simulink model "Tema_bonus_Pisai_Daria_PC1"  (R2024b)
settings: Solver=FixedStepAuto  StartTime=0.0  StopTime=1000  FixedStep=0.01  RelTol=1e-3
settings Model: Creator=dariapisai  LastModifiedBy=dariapisai

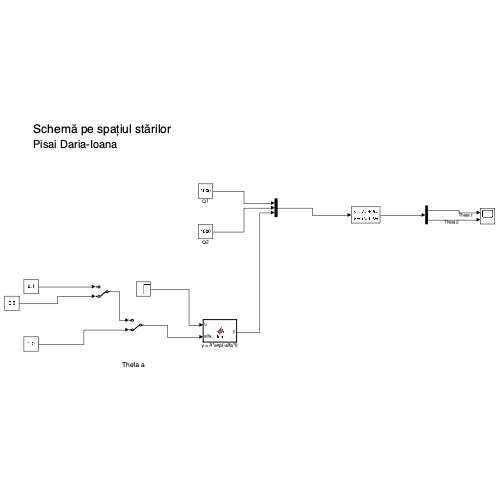
[thumbnail: Simulink's stored preview of the top-level diagram]
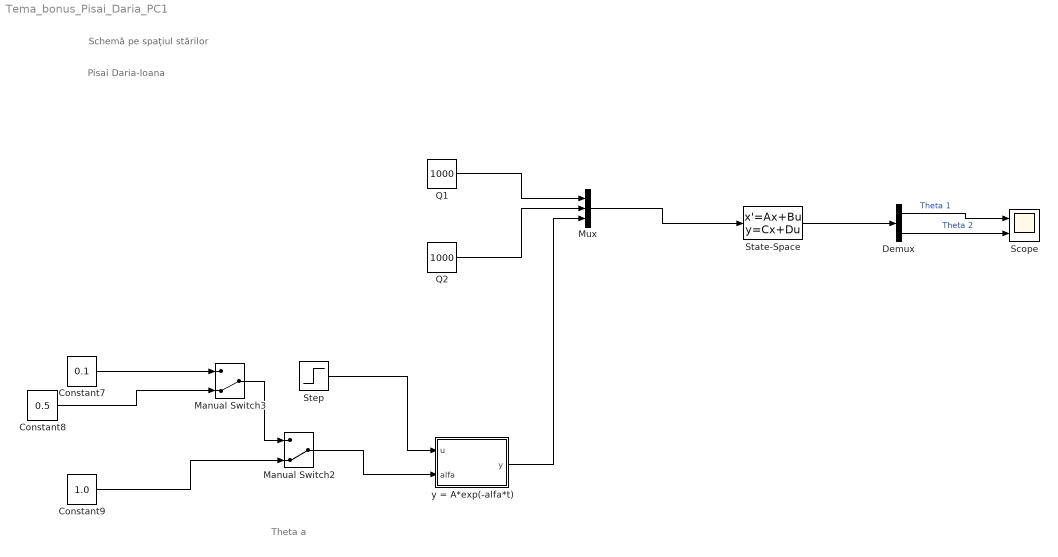
== system Tema_bonus_Pisai_Daria_PC1 ==
  note: Pisai Daria-Ioana
  note: Schemă pe spațiul stărilor
  note: Theta a
  Constant7 : Constant  Value=0.1
  Constant8 : Constant  Value=0.5
  Constant9 : Constant  Value=1.0
  Demux : Demux  Outputs=2
  Manual Switch2 : ManualSwitch  CurrentSetting=0
  Manual Switch3 : ManualSwitch  CurrentSetting=0
  Mux : Mux  Inputs=3
  Q1 : Constant  Value=1000
  Q2 : Constant  Value=1000
  Scope : Scope  NumInputPorts=2
  State-Space : StateSpace  A=[-3/625 1/1250; 1/1500 -1/1000]  B=[1/250 0 1/250; 0 1/300 1/3000]  C=[1 0; 0 1]  D=[0 0 0; 0 0 0]  InitialCondition=0
  Step : Step  Time=5  SampleTime=0
  y = A*exp(-alfa*t) : MATLAB Function  TreatAsAtomicUnit=on
  wires:
  Q1/1 -> Mux/1
  Q2/1 -> Mux/2
  Mux/1 -> State-Space/1
  Constant9/1 -> Manual Switch2/2
  Constant8/1 -> Manual Switch3/2
  Manual Switch3/1 -> Manual Switch2/1
  y = A*exp(-alfa*t)/1(y) -> Mux/3
  Manual Switch2/1 -> y = A*exp(-alfa*t)/2(alfa)
  Step/1 -> y = A*exp(-alfa*t)/1(u)
  Constant7/1 -> Manual Switch3/1
  State-Space/1 -> Demux/1
  Demux/1 -> Scope/1  "Theta 1"
  Demux/2 -> Scope/2  "Theta 2"

== matlab function Tema_bonus_Pisai_Daria_PC1/y = A*exp(-alfa*t) ==
  data: u input; y output; alfa input
function y = fcn(u, alfa)

A = 2;

y = A*exp((-alfa)*u);

end
